simulink model "tests"  (Simulink 8.0)
settings: Solver=FixedStepDiscrete  StartTime=0.0  StopTime=10  FixedStep=0.05  RelTol=1e-3
libraries: rtwinlib x1
Description:
  | Vectorized Quantizer C-MEX S-function
settings Model: Creator=The MathWorks Inc.  LastModifiedBy=x  ExtModeTrigMode=oneshot  ExtModeArmWhenConnect=off
settings SolverCC: PositivePriorityOrder=on
settings DataIOCC: LimitDataPoints=off  SignalLoggingSaveFormat=ModelDataLogs
settings OptimizationCC: BlockReduction=off  BooleanDataType=off  InitFltsAndDblsToZero=on
settings DebuggingCC: SaveWithParameterizedLinksMsg=none  SignalResolutionControl=TryResolveAllWithWarning  SolverPrmCheckMsg=none  MultiTaskDSMMsg=warning  MultiTaskCondExecSysMsg=none  FcnCallInpInsideContextMsg=UseLocalSettings
settings HardwareCC: ProdIntDivRoundTo=Zero  ProdEndianess=LittleEndian  ProdHWDeviceType=Generic->32-bit x86 compatible  TargetIntDivRoundTo=Zero  TargetEndianess=LittleEndian  TargetHWDeviceType=MATLAB Host  ProdEqTarget=off
settings SFSimCC: SimCustomHeaderCode=|
  | advapi32.dll
  | comctl32.dll
  | comdlg32.dll
  | gdi32.dll
  | kernel32.dll
  | netapi32.dll
  | shell32.dll
  | shlwapi.dll
  | user32.dll
  | WindowsCodecs.dll
settings SFSimCC: SimUserLibraries=|
  | NtDsAPI.Lib
  | NTMSAPI.Lib
  | NtQuery.Lib
  | windowscodecs.lib
settings RTWCC: ProcessScript=grt_make_rtw_hook  CustomLibrary=kernel32.lib  IncludeERTFirstTime=on  RTWCompilerOptimization=On
settings CodeAppCC: MaxIdLength=95  CustomSymbolStrType=$N$R$M_T  InternalIdentifier=Shortened

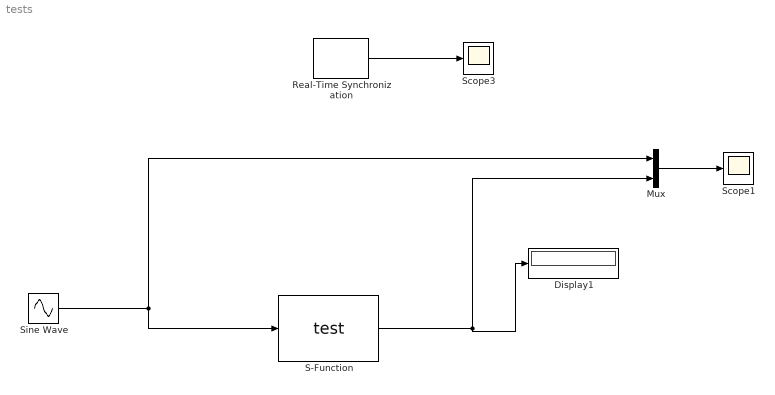
== system tests ==
  Display1 : Display
  Mux : Mux  Inputs=2
  Real-Time Synchronization : rtwinlib/Real-Time Synchronization  SampleTime=0.05  MaxMissedTicks=10000  ShowMissedTicks=on  YieldWhenWaiting=off
  S-Function : S-Function  FunctionName=test  Parameters=p1,p2  EnableBusSupport=off  mask(Serial Communication Tutorial){p1=0, p2=0}
      mask prompts: p1 "Port Name"; p2 "Baud Rate"
      mask help:
      | This Block Contains tutorial to communicate Serial Ports Through Matlab S-functions.
      |  by self-Defining the Ports. Note that To comunicate In MATLAB Real-Time Workshop
      |  Due to WATCOM Compiler for accessing Directly the Drivers independently from
      |  Windows APKs, you may need to construct the packet input/output to access Drivers
      |  In real_time Applications.
      |  Since this Method utilize the In-Time Comunication, For better Performance it's
      |  advice to close down all concurrent application in Windows Process.
      |
      |
      |   Copyright 2014 Aras Lab, K. N. Tossi university of technology, Tehran, Iran.
      |   For more Information Contact: aagand@email.kntu.ac.ir or Pedram.agand@gmail.com (@ee.kntu.ac.ir)
      mask Display:
      | port_label('input', 1, 'in')
      | port_label('output', 1, 'out')
  Scope1 : Scope
      settings: YMin=-0.5  YMax=6.5  SaveName=ScopeData2
  Scope3 : Scope
      settings: TimeRange=10  YMin=35  YMax=135
  Sine Wave : Sin  Bias=1
  wires:
  S-Function/1 -> Mux/2, Display1/1
  Mux/1 -> Scope1/1
  Real-Time Synchronization/1 -> Scope3/1
  Sine Wave/1 -> Mux/1, S-Function/1
